simulink model "BuckyWagon_01"  (Simulink 7.5)
settings: Solver=FixedStepDiscrete  StartTime=0.0  StopTime=10.0  RelTol=1e-3
PreLoadFcn:
  | try, eval([bdroot '_setup']); catch, eval('model_setup', ''); end
InitFcn:
  | try, eval([bdroot '_setup']); catch, eval('model_setup', ''); end
undefined symbols (not defined in the file or in its folder): ECU565, High, Low, miniviewSetup, motohawk_build_version, motohawk_get_faults, motohawk_setup_toolchains, motohawk_trunc_name, motohawk_vardec_config_group, motohawk_vardec_path, tc, True
libraries: MotoHawk_lib x392, simulink x29, miniview_lib x10, motohawk_control_primitives_lib x9, motohawk_engine_lib x8, MotoHawk_VDOGauge_lib x8, motohawk_annotations_lib x2
(part 2 of 7)

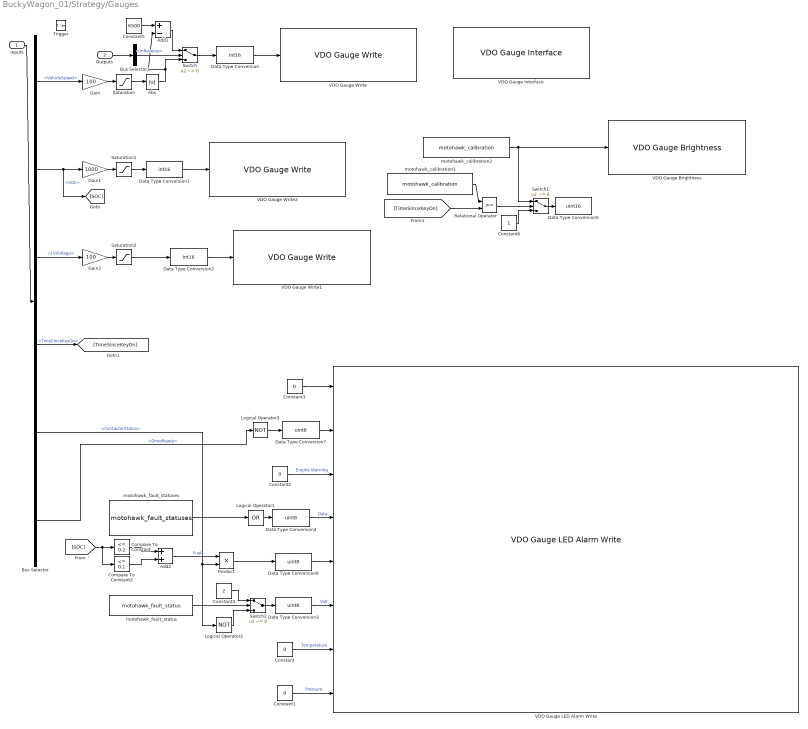
== system BuckyWagon_01/Strategy/Gauges ==
  Inputs : Inport  OutDataType=sfix(16)  OutScaling=2^0
  Outputs : Inport  Port=2  OutDataType=sfix(16)  OutScaling=2^0
  Trigger : TriggerPort  TriggerType=function-call
  Abs : Abs  OutDataType=fixdt(1, 16)  OutScaling=2^0
  Add1 : Sum  Inputs=+-  OutDataType=fixdt(1, 16)  OutScaling=2^-10
  Add2 : Sum  AccumDataTypeStr=uint8  OutDataType=fixdt(1, 16)  OutScaling=2^-10
  Bus Selector : BusSelector  OutputSignals=VehicleSpeed,SOC,LVVoltage,TimeSinceKeyOn,ContactorStatus,DriveReady
  Bus Selector1 : BusSelector  OutputSignals=InReverse
  Compare To Constant : simulink/Logic and Bit Operations/Compare To Constant  SystemSampleTime=-1  relop=<=  const=0.2  LogicOutDataTypeMode=uint8
  Compare To Constant2 : simulink/Logic and Bit Operations/Compare To Constant  SystemSampleTime=-1  relop=<=  const=0.1  LogicOutDataTypeMode=uint8
  Constant{,1..3} (4 alike) : Constant  Value=0  OutDataTypeMode=uint8  OutDataType=fixdt(1, 16)  OutScaling=2^0  OutDataTypeStr=uint8
  Constant4 : Constant  Value=2  OutDataTypeMode=uint8  OutDataType=fixdt(1, 16)  OutScaling=2^0  OutDataTypeStr=uint8
  Constant5 : Constant  Value=6500  OutDataTypeMode=int16  OutDataType=fixdt(1, 16)  OutScaling=2^0  OutDataTypeStr=int16
  Constant6 : Constant  OutDataTypeMode=int16  OutDataType=fixdt(1, 16)  OutScaling=2^0  OutDataTypeStr=int16
  Data Type Conversion : DataTypeConversion  OutDataTypeMode=int16  OutDataType=fixdt(1, 16)  OutScaling=2^0  OutDataTypeStr=int16
  Data Type Conversion1 : DataTypeConversion  OutDataTypeMode=int16  OutDataType=fixdt(1, 16)  OutScaling=2^0  OutDataTypeStr=int16
  Data Type Conversion2 : DataTypeConversion  OutDataTypeMode=int16  OutDataType=fixdt(1, 16)  OutScaling=2^0  OutDataTypeStr=int16
  Data Type Conversion{3..4,7..8} (4 alike) : DataTypeConversion  OutDataTypeMode=uint8  OutDataType=fixdt(1, 16)  OutScaling=2^0  OutDataTypeStr=uint8
  Data Type Conversion5 : DataTypeConversion  OutDataTypeMode=uint16  OutDataType=fixdt(1, 16)  OutScaling=2^0  OutDataTypeStr=uint16
  Gain : Gain  Gain=100  ParameterDataType=fixdt(1, 16)  ParameterScaling=2^0  OutDataType=fixdt(1, 16)  OutScaling=2^0
  Gain1 : Gain  Gain=1000  ParameterDataType=fixdt(1, 16)  ParameterScaling=2^0  OutDataType=fixdt(1, 16)  OutScaling=2^0
  Gain2 : Gain  Gain=100  ParameterDataType=fixdt(1, 16)  ParameterScaling=2^0  OutDataType=fixdt(1, 16)  OutScaling=2^0
  Logical Operator1 : Logic  Operator=OR  Inputs=1  AllPortsSameDT=off  OutDataTypeMode=boolean  LogicDataType=fixdt(0, 8)  OutDataTypeStr=boolean
  Logical Operator2 : Logic  Operator=NOT  Inputs=1  AllPortsSameDT=off  OutDataTypeMode=boolean  LogicDataType=fixdt(0, 8)  OutDataTypeStr=boolean
  Logical Operator3 : Logic  Operator=NOT  Inputs=1  AllPortsSameDT=off  OutDataTypeMode=boolean  LogicDataType=fixdt(0, 8)  OutDataTypeStr=boolean
  Product : Product  OutDataType=fixdt(1, 16)  OutScaling=2^0  RndMeth=Zero
  Relational Operator : RelationalOperator  LogicOutDataTypeMode=boolean  LogicDataType=fixdt(0, 8)  OutDataTypeStr=boolean
  Saturation : Saturate  UpperLimit=+10000  LowerLimit=-10000  OutDataType=fixdt(1, 16)  OutScaling=2^0
  Saturation1 : Saturate  UpperLimit=1000  LowerLimit=0  OutDataType=fixdt(1, 16)  OutScaling=2^0
  Saturation2 : Saturate  UpperLimit=2000  LowerLimit=0  OutDataType=fixdt(1, 16)  OutScaling=2^0
  Switch : Switch  Criteria=u2 ~= 0  OutDataType=fixdt(1, 16)  OutScaling=2^0
  Switch1 : Switch  Criteria=u2 ~= 0  OutDataType=fixdt(1, 16)  OutScaling=2^0
  Switch2 : Switch  Criteria=u2 ~= 0  OutDataType=fixdt(1, 16)  OutScaling=2^0
  VDO Gauge Brightness : MotoHawk_VDOGauge_lib/VDO Gauge Brightness  nam='GaugeChain'  per=2000
  VDO Gauge Interface : MotoHawk_VDOGauge_lib/VDO Gauge Interface  nam='GaugeChain'  text_resource=TACH  code_resource=NONE  val_resource=-1  target=ECU565-128  dly=1600  queue_size=128  dyn_create=off
  VDO Gauge LED Alarm Write : MotoHawk_VDOGauge_lib/VDO Gauge LED Alarm Write  nam='GaugeChain'  pri=(None)
  VDO Gauge Write : MotoHawk_VDOGauge_lib/VDO Gauge Write  nam='GaugeChain'  res=Speed  pri=(None)
  VDO Gauge Write1 : MotoHawk_VDOGauge_lib/VDO Gauge Write  nam='GaugeChain'  res=Voltage  pri=(None)
  VDO Gauge Write2 : MotoHawk_VDOGauge_lib/VDO Gauge Write  nam='GaugeChain'  res=Fuel Level  pri=(None)
  motohawk_calibration1 : MotoHawk_lib/Calibration & Probing Blocks/motohawk_calibration  nam='VDO_Gauge_StartupDelay'  val=2  storage=Calibration  show_more=on  name_source=Use Parameter  data_type=double  read_level=1  write_level=1  ovr_cals=on  view_as=Number  enum_struct={'Disabled', 'Enabled'}  vector_style=Wide Row  use_help_units=off  help=''  units=''  use_header_enum=off  row_header_enum={}  col_header_enum={}  use_min_max=off  min_val=0  max_val=7  use_precision=off  precision=''  gain=1  offset=0  exp=1  use_mototune_group=on  mototune_group='Gauges'
  motohawk_calibration2 : MotoHawk_lib/Calibration & Probing Blocks/motohawk_calibration  nam='VDO_Gauge_Brightness'  val=5  storage=Calibration  show_more=on  name_source=Use Parameter  data_type=uint16  read_level=1  write_level=1  ovr_cals=on  view_as=Number  enum_struct={'Disabled', 'Enabled'}  vector_style=Wide Row  use_help_units=off  help=''  units=''  use_header_enum=off  row_header_enum={}  col_header_enum={}  use_min_max=on  min_val=0  max_val=7  use_precision=off  precision=''  gain=1  offset=0  exp=1  use_mototune_group=on  mototune_group='Gauges'
  motohawk_fault_status : MotoHawk_lib/Fault Management Blocks/motohawk_fault_status  source=Lookup By Name  nam='GroundFlt'  status=Active
  motohawk_fault_statuses : MotoHawk_lib/Fault Management Blocks/motohawk_fault_statuses  nam=motohawk_get_faults(bdroot)  status=Active
  wires:
  Inputs/1 -> Bus Selector/1
  Bus Selector/1 -> Gain/1  "<VehicleSpeed>"
  Gain/1 -> Saturation/1
  Saturation/1 -> Abs/1
  Data Type Conversion/1 -> VDO Gauge Write/1
  Bus Selector/2 -> Gain1/1, [SOC]  "<SOC>"
  Gain1/1 -> Saturation1/1
  Saturation1/1 -> Data Type Conversion1/1
  Data Type Conversion1/1 -> VDO Gauge Write2/1
  Bus Selector/3 -> Gain2/1  "<LVVoltage>"
  Gain2/1 -> Saturation2/1
  Saturation2/1 -> Data Type Conversion2/1
  Data Type Conversion2/1 -> VDO Gauge Write1/1
  motohawk_fault_statuses/1 -> Logical Operator1/1
  Logical Operator1/1 -> Data Type Conversion4/1
  [SOC] -> Compare To Constant/1, Compare To Constant2/1
  Outputs/1 -> Bus Selector1/1
  Bus Selector1/1 -> Switch/2  "<InReverse>"
  Abs/1 -> Switch/3, Add1/2
  Switch/1 -> Data Type Conversion/1
  Constant5/1 -> Add1/1
  Add1/1 -> Switch/1
  Bus Selector/4 -> [TimeSinceKeyOn]  "<TimeSinceKeyOn>"
  [TimeSinceKeyOn] -> Relational Operator/2
  Relational Operator/1 -> Switch1/2
  Constant6/1 -> Switch1/3
  Switch1/1 -> Data Type Conversion5/1
  Bus Selector/5 -> Logical Operator2/1, Product/2  "<ContactorStatus>"
  Bus Selector/6 -> Logical Operator3/1  "<DriveReady>"
  Constant2/1 -> VDO Gauge LED Alarm Write/3  "Engine Warning"
  Data Type Conversion4/1 -> VDO Gauge LED Alarm Write/4  "Data"
  Data Type Conversion3/1 -> VDO Gauge LED Alarm Write/6  "Volt"
  Constant/1 -> VDO Gauge LED Alarm Write/7  "Temperature"
  Constant1/1 -> VDO Gauge LED Alarm Write/8  "Pressure"
  Logical Operator3/1 -> Data Type Conversion7/1
  Constant3/1 -> VDO Gauge LED Alarm Write/1
  Data Type Conversion7/1 -> VDO Gauge LED Alarm Write/2
  motohawk_calibration1/1 -> Relational Operator/1
  Data Type Conversion8/1 -> VDO Gauge LED Alarm Write/5
  Compare To Constant/1 -> Add2/1
  Compare To Constant2/1 -> Add2/2
  Product/1 -> Data Type Conversion8/1
  Add2/1 -> Product/1  "Fuel"
  motohawk_calibration2/1 -> VDO Gauge Brightness/1, Switch1/1
  motohawk_fault_status/1 -> Switch2/2
  Logical Operator2/1 -> Switch2/3
  Switch2/1 -> Data Type Conversion3/1
  Constant4/1 -> Switch2/1

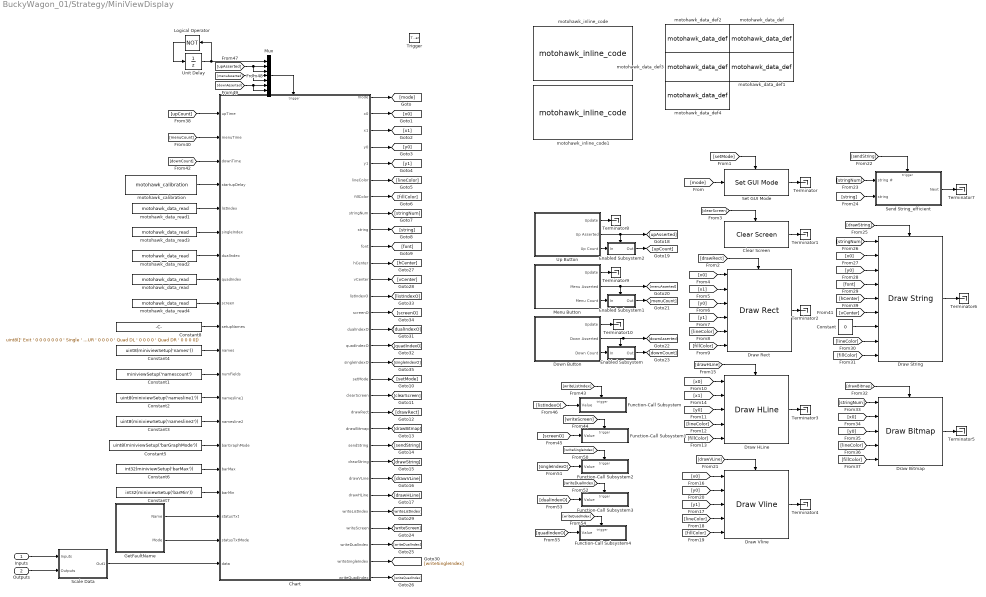
== system BuckyWagon_01/Strategy/MiniViewDisplay ==
  Inputs : Inport  OutDataType=sfix(16)  OutScaling=2^0
  Outputs : Inport  Port=2  OutDataType=sfix(16)  OutScaling=2^0
  Trigger : TriggerPort  TriggerType=function-call
  Chart : Stateflow chart  TreatAsAtomicUnit=on
      settings: RTWSystemCode=Reusable function
  Clear Screen : miniview_lib/Clear Screen  SystemSampleTime=-1  miniview_CAN_channel=1
  Constant : Constant  Value=0  OutDataType=sfix(16)  OutScaling=2^0  OutDataTypeStr=Inherit: Inherit via back propagation
  Constant1 : Constant  Value=miniviewSetup('namescount')  OutDataTypeMode=uint8  OutDataType=sfix(16)  OutScaling=2^0  OutDataTypeStr=uint8
  Constant2 : Constant  Value=uint8(miniviewSetup('namesline1'))  OutDataTypeMode=uint8  OutDataType=sfix(16)  OutScaling=2^0  OutDataTypeStr=uint8
  Constant3 : Constant  Value=uint8(miniviewSetup('namesline2'))  OutDataTypeMode=uint8  OutDataType=sfix(16)  OutScaling=2^0  OutDataTypeStr=uint8
  Constant4 : Constant  Value=uint8(miniviewSetup('names'))  OutDataTypeMode=uint8  OutDataType=sfix(16)  OutScaling=2^0  OutDataTypeStr=uint8
  Constant5 : Constant  Value=uint8(miniviewSetup('barGraphMode'))  OutDataTypeMode=uint8  OutDataType=sfix(16)  OutScaling=2^0  OutDataTypeStr=uint8
  Constant6 : Constant  Value=int32(miniviewSetup('barMax'))  OutDataTypeMode=int32  OutDataType=sfix(16)  OutScaling=2^0  OutDataTypeStr=int32
  Constant7 : Constant  Value=int32(miniviewSetup('barMin'))  OutDataTypeMode=int16  OutDataType=sfix(16)  OutScaling=2^0  OutDataTypeStr=int16
  Constant8 : Constant  Value=uint8([' Exit ' 0 0 0 0 0 0 0 ' Single ' 0 0 0 0 0 ' Dual Upper ' 0 ' Dual Lower ' 0 ' Quad UL ' 0 0 0 0 ' Quad UR ' 0 0 0 0 ' Quad DL ' 0 0 0 0 ' Quad DR ' 0 0 0 0])  OutDataTypeMode=uint8  OutDataType=sfix(16)  OutScaling=2^0  OutDataTypeStr=uint8
  Down Button : Subsystem  AncestorBlock=miniview_lib/Down Button  mask(MotoHawk MiniView Down Button){miniview_CAN_channel=1}
      mask prompts: miniview_CAN_channel "Physical CAN Channel"
      mask help: MotoHawk MiniView Down Button
      mask Display: disp(['MiniView "Down" Button\n\nChannel:  CAN_' num2str(miniview_CAN_channel)])
  Draw Bitmap : miniview_lib/Draw Bitmap  SystemSampleTime=-1  miniview_CAN_channel=1
  Draw HLine : miniview_lib/Draw HLine  SystemSampleTime=-1  miniview_CAN_channel=1
  Draw Rect : miniview_lib/Draw Rect  SystemSampleTime=-1  miniview_CAN_channel=1
  Draw String : miniview_lib/Draw String  SystemSampleTime=-1  miniview_CAN_channel=1
  Draw Vline : miniview_lib/Draw Vline  SystemSampleTime=-1  miniview_CAN_channel=1
  Enabled Subsystem : Subsystem  TreatAsAtomicUnit=on
  Enabled Subsystem1 : Subsystem  TreatAsAtomicUnit=on
  Enabled Subsystem2 : Subsystem  TreatAsAtomicUnit=on
  Function-Call Subsystem : Subsystem  TreatAsAtomicUnit=on
  Function-Call Subsystem1 : Subsystem  TreatAsAtomicUnit=on
  Function-Call Subsystem2 : Subsystem  TreatAsAtomicUnit=on
  Function-Call Subsystem3 : Subsystem  TreatAsAtomicUnit=on
  Function-Call Subsystem4 : Subsystem  TreatAsAtomicUnit=on
  GetFaultName : Subsystem
  Logical Operator : Logic  Operator=NOT  AllPortsSameDT=off  OutDataTypeMode=boolean  OutDataTypeStr=boolean
  Menu Button : Subsystem  AncestorBlock=miniview_lib/Menu Button  mask(MotoHawk MiniView Menu Button){miniview_CAN_channel=1}
      mask prompts: miniview_CAN_channel "Physical CAN Channel"
      mask help: MotoHawk MiniView Menu Button
      mask Display: disp(['MiniView "Menu" Button\n\nChannel:  CAN_' num2str(miniview_CAN_channel)])
  Mux : Mux  Inputs=7
  Scale Data : Subsystem
  Send String_efficient : Subsystem  AncestorBlock=miniview_lib/Send String  mask(MotoHawk MiniView Send String){miniview_CAN_channel=1}
      mask prompts: miniview_CAN_channel "Physical CAN Channel"
      mask help:
      | MotoHawk MiniView Send String
      |
      | Send string (#0 to #15) to gauge.
      mask Display: disp(['MiniView\nSend String\nChannel:  CAN_' num2str(miniview_CAN_channel)])
  Set GUI Mode : miniview_lib/Set GUI Mode  SystemSampleTime=-1  miniview_CAN_channel=1
  Terminator{,1..10} (11 alike) : Terminator
  Unit Delay : UnitDelay  SampleTime=-1
  Up Button : Subsystem  AncestorBlock=miniview_lib/Up Button  mask(MotoHawk MiniView Up Button){miniview_CAN_channel=1}
      mask prompts: miniview_CAN_channel "Physical CAN Channel"
      mask help: MotoHawk MiniView Up Button
      mask Display: disp(['MiniView "Up" Button\n\nChannel:  CAN_' num2str(miniview_CAN_channel)])
  motohawk_calibration : MotoHawk_lib/Calibration & Probing Blocks/motohawk_calibration  nam='startupDelay'  val=300  storage=Calibration  show_more=on  name_source=Use Parameter  data_type=uint16  read_level=1  write_level=1  ovr_cals=on  view_as=Number  enum_struct={'Disabled', 'Enabled'}  vector_style=Wide Row  use_help_units=on  help='Time to wait before drawing on the miniview.'  units='s'  use_header_enum=off  row_header_enum={}  col_header_enum={}  use_min_max=on  min_val=0  max_val=10  use_precision=on  precision='1.3'  gain=0.005  offset=0  exp=1  use_mototune_group=off  mototune_group=motohawk_vardec_path(gcb)
  motohawk_data_def : MotoHawk_lib/Data Storage Blocks/motohawk_data_def  nam='quadIndex'  container_nam=''  data=[0 5 16 19]  typ=uint8  struct_nam='MyStruct'  storage=NonVolatile  outputRef=off  use_vardec=on  window=Display  read_level=1  write_level=1  ovr_cals=on  view_as=Number  enum_struct={'Disabled', 'Enabled'}  vector_style=Tall Column  use_help_units=on  help=''  units=''  use_header_enum=off  row_header_enum=''  col_header_enum=''  use_min_max=off  min_val=-inf  max_val=inf  use_precision=off  precision=''  gain=1  offset=0  exp=1  use_mototune_group=off  mototune_group=motohawk_vardec_path(gcb)  eval_name=quadIndex  data_stores=motohawk_sfun_data_def_data_stores  struct_instances=motohawk_sfun_data_def_struct_instances  vardecs=motohawk_sfun_data_def_vardecs
  motohawk_data_def1 : MotoHawk_lib/Data Storage Blocks/motohawk_data_def  nam='listIndex'  container_nam=''  data=0  typ=uint8  struct_nam='MyStruct'  storage=NonVolatile  outputRef=off  use_vardec=on  window=Display  read_level=1  write_level=1  ovr_cals=on  view_as=Number  enum_struct={'Disabled', 'Enabled'}  vector_style=Tall Column  use_help_units=on  help=''  units=''  use_header_enum=off  row_header_enum=''  col_header_enum=''  use_min_max=off  min_val=-inf  max_val=inf  use_precision=off  precision=''  gain=1  offset=0  exp=1  use_mototune_group=off  mototune_group=motohawk_vardec_path(gcb)  eval_name=listIndex  data_stores=motohawk_sfun_data_def_data_stores  struct_instances=motohawk_sfun_data_def_struct_instances  vardecs=motohawk_sfun_data_def_vardecs
  motohawk_data_def2 : MotoHawk_lib/Data Storage Blocks/motohawk_data_def  nam='dualIndex'  container_nam=''  data=[10 27]  typ=uint8  struct_nam='MyStruct'  storage=NonVolatile  outputRef=off  use_vardec=on  window=Display  read_level=1  write_level=1  ovr_cals=on  view_as=Number  enum_struct={'Disabled', 'Enabled'}  vector_style=Tall Column  use_help_units=on  help=''  units=''  use_header_enum=off  row_header_enum=''  col_header_enum=''  use_min_max=off  min_val=-inf  max_val=inf  use_precision=off  precision=''  gain=1  offset=0  exp=1  use_mototune_group=off  mototune_group=motohawk_vardec_path(gcb)  eval_name=dualIndex  data_stores=motohawk_sfun_data_def_data_stores  struct_instances=motohawk_sfun_data_def_struct_instances  vardecs=motohawk_sfun_data_def_vardecs
  motohawk_data_def3 : MotoHawk_lib/Data Storage Blocks/motohawk_data_def  nam='singleIndex'  container_nam=''  data=15  typ=uint8  struct_nam='MyStruct'  storage=NonVolatile  outputRef=off  use_vardec=on  window=Display  read_level=1  write_level=1  ovr_cals=on  view_as=Number  enum_struct={'Disabled', 'Enabled'}  vector_style=Tall Column  use_help_units=on  help=''  units=''  use_header_enum=off  row_header_enum=''  col_header_enum=''  use_min_max=off  min_val=-inf  max_val=inf  use_precision=off  precision=''  gain=1  offset=0  exp=1  use_mototune_group=off  mototune_group=motohawk_vardec_path(gcb)  eval_name=singleIndex  data_stores=motohawk_sfun_data_def_data_stores  struct_instances=motohawk_sfun_data_def_struct_instances  vardecs=motohawk_sfun_data_def_vardecs
  motohawk_data_def4 : MotoHawk_lib/Data Storage Blocks/motohawk_data_def  nam='screen'  container_nam=''  data=0  typ=uint8  struct_nam='MyStruct'  storage=NonVolatile  outputRef=off  use_vardec=on  window=Display  read_level=1  write_level=1  ovr_cals=on  view_as=Number  enum_struct={'Disabled', 'Enabled'}  vector_style=Tall Column  use_help_units=on  help=''  units=''  use_header_enum=off  row_header_enum=''  col_header_enum=''  use_min_max=off  min_val=-inf  max_val=inf  use_precision=off  precision=''  gain=1  offset=0  exp=1  use_mototune_group=off  mototune_group=motohawk_vardec_path(gcb)  eval_name=screen  data_stores=motohawk_sfun_data_def_data_stores  struct_instances=motohawk_sfun_data_def_struct_instances  vardecs=motohawk_sfun_data_def_vardecs
  motohawk_data_read : MotoHawk_lib/Data Storage Blocks/motohawk_data_read  source=Lookup By Name  structure=Vector  operation=Read entire data structure at once  sz_vec=4  sz_row=2  sz_col=3  typ=uint8  nam='quadIndex'  checkNull=on  struct_inst_name='Struct1'  struct_nam='MyStruct'
  motohawk_data_read1 : MotoHawk_lib/Data Storage Blocks/motohawk_data_read  source=Lookup By Name  structure=Scalar  operation=Read scalar from location by index  sz_vec=4  sz_row=2  sz_col=3  typ=uint8  nam='listIndex'  checkNull=on  struct_inst_name='Struct1'  struct_nam='MyStruct'
  motohawk_data_read2 : MotoHawk_lib/Data Storage Blocks/motohawk_data_read  source=Lookup By Name  structure=Vector  operation=Read entire data structure at once  sz_vec=2  sz_row=2  sz_col=3  typ=uint8  nam='dualIndex'  checkNull=on  struct_inst_name='Struct1'  struct_nam='MyStruct'
  motohawk_data_read3 : MotoHawk_lib/Data Storage Blocks/motohawk_data_read  source=Lookup By Name  structure=Scalar  operation=Read scalar from location by index  sz_vec=4  sz_row=2  sz_col=3  typ=uint8  nam='singleIndex'  checkNull=on  struct_inst_name='Struct1'  struct_nam='MyStruct'
  motohawk_data_read4 : MotoHawk_lib/Data Storage Blocks/motohawk_data_read  source=Lookup By Name  structure=Scalar  operation=Read entire data structure at once  sz_vec=4  sz_row=2  sz_col=3  typ=uint8  nam='screen'  checkNull=on  struct_inst_name='Struct1'  struct_nam='MyStruct'
  motohawk_inline_code : MotoHawk_lib/Extra Development Blocks/motohawk_inline_code  include_code='#include <stdio.h>'  start_code=''  output_code=''
  motohawk_inline_code1 : MotoHawk_lib/Extra Development Blocks/motohawk_inline_code  include_code='#define charPtr(p) ((char*)p)'  start_code=''  output_code=''
  wires:
  Outputs/1 -> Scale Data/2(Outputs)
  Inputs/1 -> Scale Data/1(Inputs)
  Chart/1(mode) -> [mode]
  Chart/2(x0) -> [x0]
  Chart/3(x1) -> [x1]
  Chart/4(y0) -> [y0]
  Chart/5(y1) -> [y1]
  Chart/6(lineColor) -> [lineColor]
  Chart/7(fillColor) -> [fillColor]
  Chart/8(stringNum) -> [stringNum]
  Chart/9(string) -> [string]
  Chart/10(font) -> [font]
  Chart/19(clearScreen) -> [clearScreen]
  Chart/20(drawRect) -> [drawRect]
  Chart/21(drawBitmap) -> [drawBitmap]
  Chart/22(sendString) -> [sendString]
  Chart/23(drawString) -> [drawString]
  Chart/24(drawVLine) -> [drawVLine]
  Chart/25(drawHLine) -> [drawHLine]
  [setMode] -> Set GUI Mode/Trigger
  [mode] -> Set GUI Mode/1
  Set GUI Mode/1 -> Terminator/1
  [clearScreen] -> Clear Screen/Trigger
  Clear Screen/1 -> Terminator1/1
  [drawRect] -> Draw Rect/Trigger
  [x0] -> Draw Rect/1
  [x1] -> Draw Rect/2
  [y0] -> Draw Rect/3
  [y1] -> Draw Rect/4
  [lineColor] -> Draw Rect/5
  [fillColor] -> Draw Rect/6
  [x0] -> Draw HLine/1
  [x1] -> Draw HLine/2
  [y0] -> Draw HLine/3
  [lineColor] -> Draw HLine/4
  [fillColor] -> Draw HLine/5
  [drawHLine] -> Draw HLine/Trigger
  [x0] -> Draw Vline/1
  [y0] -> Draw Vline/2
  [y1] -> Draw Vline/3
  [lineColor] -> Draw Vline/4
  [fillColor] -> Draw Vline/5
  [drawVLine] -> Draw Vline/Trigger
  Draw Rect/1 -> Terminator2/1
  Draw Vline/1 -> Terminator4/1
  Draw HLine/1 -> Terminator3/1
  [sendString] -> Send String_efficient/Trigger
  [stringNum] -> Send String_efficient/1(string #)
  [string] -> Send String_efficient/2(string)
  [drawString] -> Draw String/Trigger
  [stringNum] -> Draw String/1
  [x0] -> Draw String/2
  [y0] -> Draw String/3
  [font] -> Draw String/4
  [lineColor] -> Draw String/8
  [fillColor] -> Draw String/9
  [drawBitmap] -> Draw Bitmap/Trigger
  [stringNum] -> Draw Bitmap/1
  [x0] -> Draw Bitmap/2
  [y0] -> Draw Bitmap/3
  [lineColor] -> Draw Bitmap/4
  [fillColor] -> Draw Bitmap/5
  Draw Bitmap/1 -> Terminator5/1
  Draw String/1 -> Terminator6/1
  Send String_efficient/1(Next) -> Terminator7/1
  [upCount] -> Chart/1(upTime)
  [menuCount] -> Chart/2(menuTime)
  [downCount] -> Chart/3(downTime)
  Up Button/2(Up Asserted) -> [upAsserted], Enabled Subsystem2/Enable
  Down Button/2(Down Asserted) -> [downAsserted], Enabled Subsystem/Enable
  Menu Button/2(Menu Asserted) -> [menuAsserted], Enabled Subsystem1/Enable
  [upAsserted] -> Mux/2, Mux/3
  [menuAsserted] -> Mux/4, Mux/5
  [downAsserted] -> Mux/6, Mux/7
  Mux/1 -> Chart/Trigger
  Constant/1 -> Draw String/7
  [hCenter] -> Draw String/5
  [vCenter] -> Draw String/6
  Chart/11(hCenter) -> [hCenter]
  Chart/12(vCenter) -> [vCenter]
  Unit Delay/1 -> Mux/1, Logical Operator/1
  Constant4/1 -> Chart/11(names)
  Logical Operator/1 -> Unit Delay/1
  Scale Data/1(Out1) -> Chart/20(data)
  Constant2/1 -> Chart/13(namesline1)
  Constant3/1 -> Chart/14(namesline2)
  motohawk_data_read1/1 -> Chart/5(listIndex)
  motohawk_data_read/1 -> Chart/8(quadIndex)
  Chart/26(writeListIndex) -> [writeListIndex]
  [writeListIndex] -> Function-Call Subsystem/Trigger
  motohawk_data_read2/1 -> Chart/7(dualIndex)
  motohawk_data_read3/1 -> Chart/6(singleIndex)
  Constant5/1 -> Chart/15(barGraphMode)
  Constant6/1 -> Chart/16(barMax)
  Constant7/1 -> Chart/17(barMin)
  Up Button/1(Update) -> Terminator8/1
  Menu Button/1(Update) -> Terminator9/1
  Down Button/1(Update) -> Terminator10/1
  Constant8/1 -> Chart/10(setupNames)
  Chart/27(writeScreen) -> [writeScreen]
  [writeScreen] -> Function-Call Subsystem1/Trigger
  motohawk_data_read4/1 -> Chart/9(screen)
  Down Button/3(Down Count) -> Enabled Subsystem/1(In)
  Enabled Subsystem/1(Out) -> [downCount]
  Menu Button/3(Menu Count) -> Enabled Subsystem1/1(In)
  Enabled Subsystem1/1(Out) -> [menuCount]
  Up Button/3(Up Count) -> Enabled Subsystem2/1(In)
  Enabled Subsystem2/1(Out) -> [upCount]
  Chart/28(writeDualIndex) -> [writeDualIndex]
  Chart/29(writeSingleIndex) -> [writeSingleIndex]
  Chart/30(writeQuadIndex) -> [writeQuadIndex]
  Chart/13(listIndexO) -> [listIndexO]
  Chart/14(screenO) -> [screenO]
  Chart/15(dualIndexO) -> [dualIndexO]
  Chart/16(quadIndexO) -> [quadIndexO]
  Chart/17(singleIndexO) -> [singleIndexO]
  [screenO] -> Function-Call Subsystem1/1(Value)
  [listIndexO] -> Function-Call Subsystem/1(Value)
  [writeSingleIndex] -> Function-Call Subsystem2/Trigger
  [singleIndexO] -> Function-Call Subsystem2/1(Value)
  [writeDualIndex] -> Function-Call Subsystem3/Trigger
  [dualIndexO] -> Function-Call Subsystem3/1(Value)
  [writeQuadIndex] -> Function-Call Subsystem4/Trigger
  [quadIndexO] -> Function-Call Subsystem4/1(Value)
  Constant1/1 -> Chart/12(numFields)
  Chart/18(setMode) -> [setMode]
  GetFaultName/1(Name) -> Chart/18(statusTxt)
  GetFaultName/2(Mode) -> Chart/19(statusTxtMode)
  motohawk_calibration/1 -> Chart/4(startupDelay)
